simulink model "orbit_sim"  (R2025b)
settings: Solver=ode45  StartTime=0.0  StopTime=T_sim  MaxStep=10  RelTol=1e-8  AbsTol=1e-9
undefined symbols (not defined in the file or in its folder): F_ext, state0
settings Model: Creator=Kang  LastModifiedBy=Kang

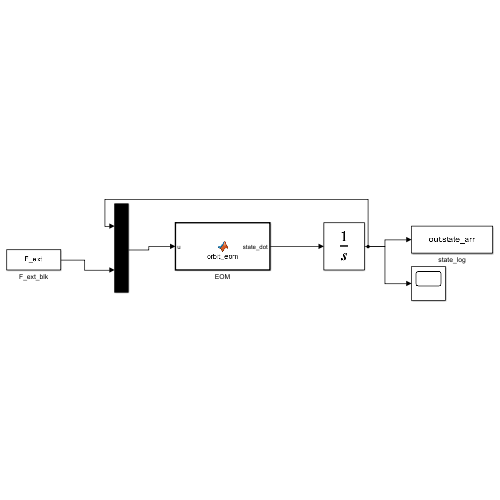
[thumbnail: Simulink's stored preview of the top-level diagram]
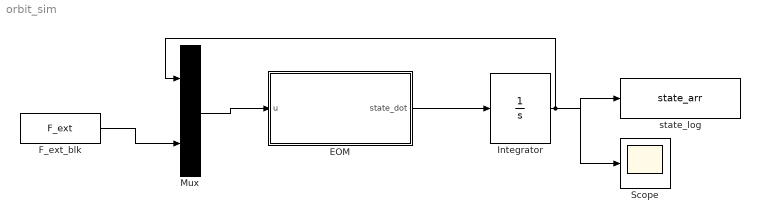
== system orbit_sim ==
  EOM : MATLAB Function  TreatAsAtomicUnit=on
  F_ext_blk : Constant  Value=F_ext  OutDataTypeStr=double
  Integrator : Integrator  InitialCondition=state0
  Mux : Mux  Inputs=2
  Scope : Scope
  state_log : ToWorkspace  VariableName=state_arr  SampleTime=-1
  wires:
  Integrator/1 -> Mux/1, state_log/1, Scope/1
  F_ext_blk/1 -> Mux/2
  Mux/1 -> EOM/1(u)
  EOM/1(state_dot) -> Integrator/1

== matlab function orbit_sim/EOM ==
  data: u input; state_dot output
function state_dot = orbit_eom(u)
%#codegen
% u = [x;y;z;vx;vy;vz;Fx;Fy;Fz]  (9×1)
% state_dot = [vx;vy;vz;ax;ay;az] (6×1)
GM_c = 3.986004418e14;
m_c  = 500;
pos  = u(1:3);
vel  = u(4:6);
Fext = u(7:9);
r3   = norm(pos)^3;
acc  = -(GM_c / r3) .* pos + Fext ./ m_c;
state_dot = [vel; acc];
